simulink model "InverseTimeConstant_TestModel"  (R2014a)
settings: Solver=ode45  StartTime=0.0  StopTime=10.0  RelTol=1e-3
libraries: rocket_angular_flight_library x1
settings Model: Creator=scorpii  LastModifiedBy=scorpii

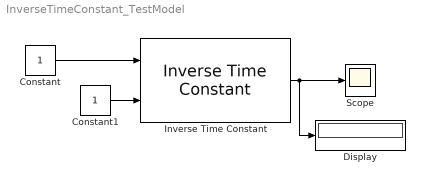
== system InverseTimeConstant_TestModel ==
  Constant : Constant
  Constant1 : Constant
  Display : Display
  Inverse Time Constant : rocket_angular_flight_library/Inverse Time Constant
  Scope : Scope
  wires:
  Inverse Time Constant/1 -> Display/1, Scope/1
  Constant/1 -> Inverse Time Constant/1
  Constant1/1 -> Inverse Time Constant/2
